simulink model "ClassDMain"  (R2020a)
settings: Solver=VariableStepAuto  StartTime=0.0  StopTime=1  MaxStep=1e-5  RelTol=1e-3
libraries: powerlib x33, dsparch4 x6, powerlib_meascontrol x6, simulink x2
settings Model: Creator=burmesdani  LastModifiedBy=Keshav
settings SolverCC: ZeroCrossAlgorithm=Adaptive
settings DataIOCC: ReturnWorkspaceOutputs=off
settings DebuggingCC: IgnoredZcDiagnostic=none  ArithmeticOperatorsInVariantConditions=warning
settings SFSimCC: SimUseLocalCustomCode=off  CustomCodeUndefinedFunction=UseInterfaceOnly
settings RTWCC: RTWUseLocalCustomCode=off

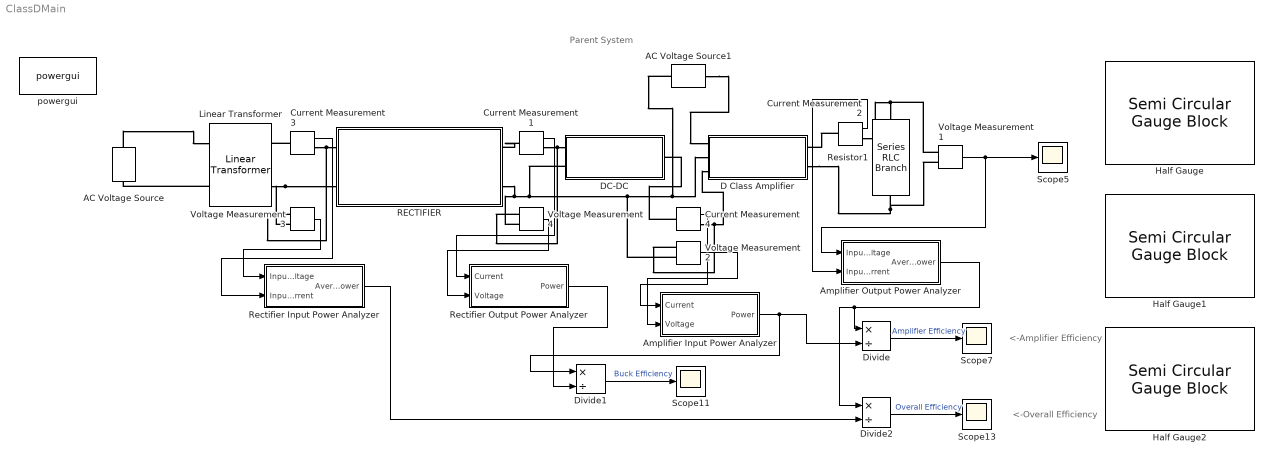
== system ClassDMain ==
  note: Parent System
  note: <-Overall Efficiency
  note: <-Amplifier Efficiency
  AC Voltage Source : powerlib/Electrical Sources/AC Voltage Source  Amplitude=240*sqrt(2)  Phase=0  Frequency=50  SampleTime=0  Measurements=None  BusType=swing  Pref=10e3  Qref=0  Qmin=-inf  Qmax=+inf
  AC Voltage Source1 : powerlib/Electrical Sources/AC Voltage Source  Amplitude=1  Phase=0  Frequency=100  SampleTime=0  Measurements=None  BusType=swing  Pref=10e3  Qref=0  Qmin=-inf  Qmax=+inf
  Amplifier Input Power Analyzer : Subsystem
  Amplifier Output Power Analyzer : Subsystem
  Current Measurement{1..4} (4 alike) : powerlib/Measurements/Current Measurement  PhasorSimulation=off  OutputType=Complex  PSBequivalent=0
  D Class Amplifier : Subsystem  mask{mxsw=1, Fts=2000}
      mask prompts: mxsw "Max input swing"; Fts "Switching Freq"
  DC-DC : Subsystem  mask{Fts=40000, opv=26}
      mask prompts: Fts "SwitchingFreq"; opv "OutputVoltage"
  Divide : Product  Inputs=*/
  Divide1 : Product  Inputs=*/
  Divide2 : Product  Inputs=*/
  Half Gauge : SemiCircularGaugeBlock  ScaleMax=1
  Half Gauge1 : SemiCircularGaugeBlock  ScaleMax=1
  Half Gauge2 : SemiCircularGaugeBlock  ScaleMax=1
  Linear Transformer : powerlib/Elements/Linear Transformer  UNITS=pu  NominalPower=[ 250e6 60 ]  winding1="[ 240  0.002  0.08 ]"  winding2="[ 60  0.002  0.08 ]"  ThreeWindings=off  winding3=[ 315e3 0.002 0.08 ]  RmLm=[ 500 500 ]  Measurements=None  DataType=off
  RECTIFIER : Subsystem
  Rectifier Input Power Analyzer : Subsystem
  Rectifier Output Power Analyzer : Subsystem
  Resistor1 : powerlib/Elements/Series RLC Branch  LConnTagsString=__new0  RConnTagsString=__new0  BranchType=R  Resistance=4  Inductance=1e-3  SetiL0=off  InitialCurrent=0  Capacitance=100e-6  Setx0=off  InitialVoltage=0  Measurements=None
  Scope{5,7,11,13} (4 alike) : Scope
  Voltage Measurement{1..4} (4 alike) : powerlib/Measurements/Voltage Measurement  PhasorSimulation=off  OutputType=Magnitude  PSBequivalent=0
  powergui : powerlib/powergui  Priority=1  SimulationMode=Continuous  SampleTime=50e-6  frequency=60  Iterations=50  frequencyindice=100  Pbase=100e6  ErrMax=1e-4  UnitsV=kV  UnitsW=MW  buscounter=0  FunctionMessages=off  echomessages=off  EnableUseOfTLC=off  CurrentSourceSwitches=off  DisableSnubberDevices=off  DisableRonSwitches=off  DisableVfSwitches=off  DisplayEquations=off  AutomaticDiscreteSolvers=off  SolverType=Tustin/Backward Euler (TBE)  Interpol=off  ExternalGateDelay=off  methode=off  Ts=100  x0status=blocks  SPID=on  SwTol=0  HookPort=off  NonlinearTolerance=1e-4  nMaxIteration=100  ContinueOnMaxIteration=off  RestoreLinks=warning  ResistiveCurrentMeasurement=off  Frange=[0:2:500]  Ylog=off  Xlog=on  ShowGrid=off  save=off  variable=ZData  structure=0  ZoomFFT=off  StartTime=0.0  cycles=1  DisplayStyle=1  fundamental=60  FreqAxis=off  MaxFrequency=1000  frequencyindicesteady=1  RmsSteady=1  display=off
  wires:
  Divide/1 -> Scope7/1  "Amplifier Efficiency"
  Divide1/1 -> Scope11/1  "Buck Efficiency"
  Divide2/1 -> Scope13/1  "Overall Efficiency"
  Voltage Measurement3/1 -> Rectifier Input Power Analyzer/1(Input Voltage)
  Current Measurement3/1 -> Rectifier Input Power Analyzer/2(Input Current)
  Current Measurement1/1 -> Rectifier Output Power Analyzer/1(Current)
  Voltage Measurement4/1 -> Rectifier Output Power Analyzer/2(Voltage)
  Current Measurement4/1 -> Amplifier Input Power Analyzer/1(Current)
  Voltage Measurement2/1 -> Amplifier Input Power Analyzer/2(Voltage)
  Voltage Measurement1/1 -> Scope5/1, Amplifier Output Power Analyzer/1(Input Voltage)
  Current Measurement2/1 -> Amplifier Output Power Analyzer/2(Input Current)
  Rectifier Input Power Analyzer/1(Average power) -> Divide2/2
  Amplifier Output Power Analyzer/1(Average power) -> Divide/1, Divide2/1
  Amplifier Input Power Analyzer/1(Power) -> Divide1/1, Divide/2
  Rectifier Output Power Analyzer/1(Power) -> Divide1/2
  connections:
  Linear Transformer/RConn2 -- RECTIFIER/LConn2 -- Voltage Measurement3/LConn2
  Linear Transformer/LConn2 -- AC Voltage Source/LConn1
  AC Voltage Source/RConn1 -- Linear Transformer/LConn1
  RECTIFIER/RConn2 -- D Class Amplifier/LConn2 -- AC Voltage Source1/LConn1 -- Voltage Measurement2/LConn2 -- DC-DC/LConn2 -- Voltage Measurement4/LConn2
  Current Measurement1/RConn1 -- Voltage Measurement4/LConn1 -- DC-DC/LConn1
  Current Measurement1/LConn1 -- RECTIFIER/RConn1
  AC Voltage Source1/RConn1 -- D Class Amplifier/LConn1
  D Class Amplifier/RConn2 -- Voltage Measurement1/LConn2 -- Resistor1/RConn1
  Current Measurement2/LConn1 -- D Class Amplifier/RConn1
  Current Measurement2/RConn1 -- Voltage Measurement1/LConn1 -- Resistor1/LConn1
  Current Measurement4/RConn1 -- Voltage Measurement2/LConn1 -- D Class Amplifier/LConn3
  Current Measurement4/LConn1 -- DC-DC/RConn1
  Current Measurement3/LConn1 -- Linear Transformer/RConn1
  Current Measurement3/RConn1 -- Voltage Measurement3/LConn1 -- RECTIFIER/LConn1

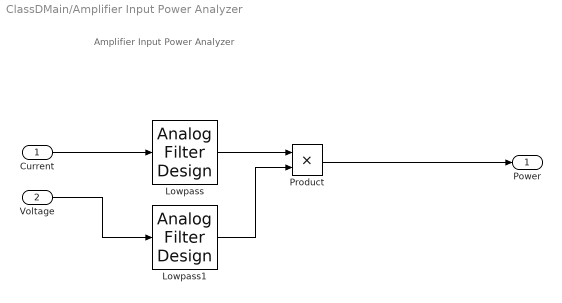
== system ClassDMain/Amplifier Input Power Analyzer ==
  note: Amplifier Input Power Analyzer
  Current : Inport
  Voltage : Inport  Port=2
  Lowpass : dsparch4/Analog Filter Design  method=Butterworth  filttype=Lowpass  N=8  Wlo=200  Whi=80  Rp=1  Rs=40
  Lowpass1 : dsparch4/Analog Filter Design  method=Butterworth  filttype=Lowpass  N=8  Wlo=200  Whi=80  Rp=1  Rs=40
  Product : Product
  Power : Outport
  wires:
  Current/1 -> Lowpass/1
  Lowpass/1 -> Product/1
  Product/1 -> Power/1
  Lowpass1/1 -> Product/2
  Voltage/1 -> Lowpass1/1

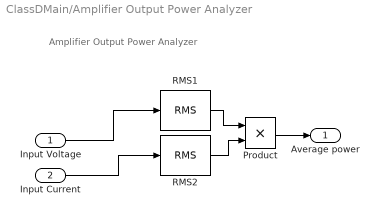
== system ClassDMain/Amplifier Output Power Analyzer ==
  note: Amplifier Output Power Analyzer
  Input Voltage : Inport
  Input Current : Inport  Port=2
  Product : Product
  RMS1 : powerlib_meascontrol/Measurements/RMS  TrueRMS=on  Freq=200  RMSInit=0  Ts=0
  RMS2 : powerlib_meascontrol/Measurements/RMS  TrueRMS=on  Freq=200  RMSInit=0  Ts=0
  Average power : Outport
  wires:
  Product/1 -> Average power/1
  Input Voltage/1 -> RMS1/1
  RMS1/1 -> Product/1
  RMS2/1 -> Product/2
  Input Current/1 -> RMS2/1

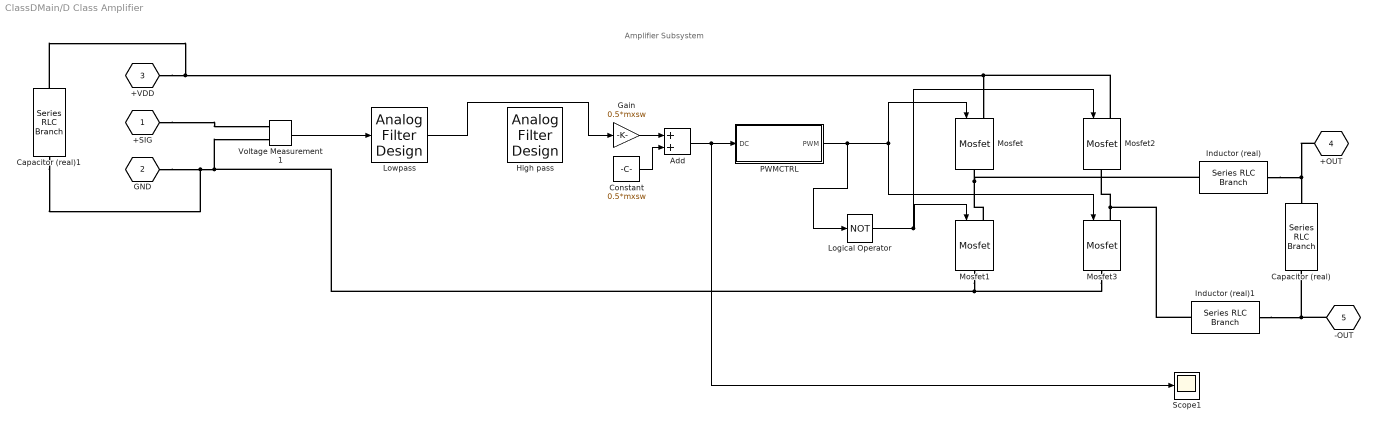
== system ClassDMain/D Class Amplifier ==
  note: Amplifier Subsystem
  Add : Sum
  Capacitor (real) : powerlib/Elements/Series RLC Branch  LConnTagsString=__new0  RConnTagsString=__new0  BranchType=RC  Resistance=0.2  Inductance=1e-3  SetiL0=off  InitialCurrent=0  Capacitance=160e-6  Setx0=off  InitialVoltage=0  Measurements=None
  Capacitor (real)1 : powerlib/Elements/Series RLC Branch  LConnTagsString=__new0  RConnTagsString=__new0  BranchType=RC  Resistance=0.2  Inductance=1e-3  SetiL0=off  InitialCurrent=0  Capacitance=4.7e-3  Setx0=off  InitialVoltage=0  Measurements=None
  Constant : Constant  Value=0.5*mxsw
  Gain : Gain  Gain=0.5*mxsw
  High pass : dsparch4/Analog Filter Design  method=Chebyshev I  filttype=Highpass  N=8  Wlo=31.4  Whi=80  Rp=1  Rs=40
  Inductor (real) : powerlib/Elements/Series RLC Branch  LConnTagsString=__new0  RConnTagsString=__new0  BranchType=RL  Resistance=0.08  Inductance=1e-3  SetiL0=off  InitialCurrent=0  Capacitance=10e-6  Setx0=off  InitialVoltage=0  Measurements=None
  Inductor (real)1 : powerlib/Elements/Series RLC Branch  LConnTagsString=__new0  RConnTagsString=__new0  BranchType=RL  Resistance=0.08  Inductance=1e-3  SetiL0=off  InitialCurrent=0  Capacitance=10e-6  Setx0=off  InitialVoltage=0  Measurements=None
  Logical Operator : Logic  Operator=NOT  Inputs=1  IconShape=distinctive  AllPortsSameDT=off  OutDataTypeStr=boolean
  Lowpass : dsparch4/Analog Filter Design  method=Chebyshev I  filttype=Lowpass  N=8  Wlo=3000  Whi=80  Rp=1  Rs=40
  Mosfet{,1..3} (4 alike) : powerlib/Power Electronics/Mosfet  Ron=0.1  Lon=0  Rd=0.01  Vfd=0  IC=0  Rs=1e5  Cs=inf  Measurements=off
  PWMCTRL : Subsystem  mask{Ft=Fts}
      mask prompts: Ft "Switching Freq"
  Scope1 : Scope
  Voltage Measurement1 : powerlib/Measurements/Voltage Measurement  PhasorSimulation=off  OutputType=Magnitude  PSBequivalent=0
      link override source: GotoTag=T38_3671_2614244151095
  +SIG : PMIOPort  Tag=PMCPort  Side=Left
  GND : PMIOPort  Tag=PMCPort  Port=2  Side=Left
  +VDD : PMIOPort  Tag=PMCPort  Port=3  Side=Left
  +OUT : PMIOPort  Tag=PMCPort  Port=4  Side=Right
  -OUT : PMIOPort  Tag=PMCPort  Port=5  Side=Right
  wires:
  Voltage Measurement1/1 -> Lowpass/1
  Gain/1 -> Add/1
  Constant/1 -> Add/2
  Add/1 -> Scope1/1, PWMCTRL/1(DC)
  PWMCTRL/1(PWM) -> Logical Operator/1, Mosfet3/1, Mosfet/1
  Logical Operator/1 -> Mosfet2/1, Mosfet1/1
  Lowpass/1 -> Gain/1
  connections:
  +SIG/RConn1 -- Voltage Measurement1/LConn1
  GND/RConn1 -- Mosfet3/RConn1 -- Mosfet1/RConn1 -- Voltage Measurement1/LConn2 -- Capacitor (real)1/RConn1
  +VDD/RConn1 -- Capacitor (real)1/LConn1 -- Mosfet2/LConn1 -- Mosfet/LConn1
  Mosfet1/LConn1 -- Inductor (real)/RConn1 -- Mosfet/RConn1
  Mosfet3/LConn1 -- Mosfet2/RConn1 -- Inductor (real)1/RConn1
  Inductor (real)/LConn1 -- Capacitor (real)/LConn1 -- +OUT/RConn1
  -OUT/RConn1 -- Inductor (real)1/LConn1 -- Capacitor (real)/RConn1

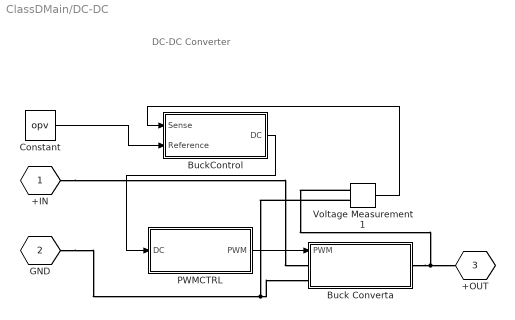
== system ClassDMain/DC-DC ==
  note: DC-DC Converter
  Buck Converta : Subsystem
  BuckControl : Subsystem
  Constant : Constant  Value=opv
  PWMCTRL : Subsystem  mask{Ft=Fts}
      mask prompts: Ft "Switching Freq"
  Voltage Measurement1 : powerlib/Measurements/Voltage Measurement  PhasorSimulation=off  OutputType=Magnitude  PSBequivalent=0
  +IN : PMIOPort  Tag=PMCPort  Side=Left
  GND : PMIOPort  Tag=PMCPort  Port=2  Side=Left
  +OUT : PMIOPort  Tag=PMCPort  Port=3  Side=Right
  wires:
  PWMCTRL/1(PWM) -> Buck Converta/1(PWM)
  BuckControl/1(DC) -> PWMCTRL/1(DC)
  Constant/1 -> BuckControl/2(Reference)
  Voltage Measurement1/1 -> BuckControl/1(Sense)
  connections:
  +IN/RConn1 -- Buck Converta/LConn1
  GND/RConn1 -- Voltage Measurement1/LConn2 -- Buck Converta/LConn2
  Buck Converta/RConn1 -- Voltage Measurement1/LConn1 -- +OUT/RConn1

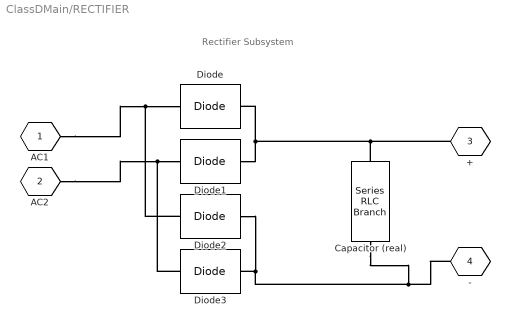
== system ClassDMain/RECTIFIER ==
  note: Rectifier Subsystem
  Capacitor (real) : powerlib/Elements/Series RLC Branch  LConnTagsString=__new0  RConnTagsString=__new0  BranchType=RC  Resistance=0.05  Inductance=1e-3  SetiL0=off  InitialCurrent=0  Capacitance=10e-3  Setx0=off  InitialVoltage=0  Measurements=None
  Diode{,1..3} (4 alike) : powerlib/Power Electronics/Diode  Ron=0.001  Lon=0  Vf=0.8  IC=0  UseSnubber=0  Rs=500  Cs=250e-9  Measurements=off
  AC1 : PMIOPort  Tag=PMCPort  Side=Left
  AC2 : PMIOPort  Tag=PMCPort  Port=2  Side=Left
  + : PMIOPort  Tag=PMCPort  Port=3  Side=Right
  - : PMIOPort  Tag=PMCPort  Port=4  Side=Right
  connections:
  AC1/RConn1 -- Diode2/RConn1 -- Diode/LConn1
  AC2/RConn1 -- Diode3/RConn1 -- Diode1/LConn1
  Diode1/RConn1 -- +/RConn1 -- Capacitor (real)/LConn1 -- Diode/RConn1
  Diode2/LConn1 -- Capacitor (real)/RConn1 -- -/RConn1 -- Diode3/LConn1

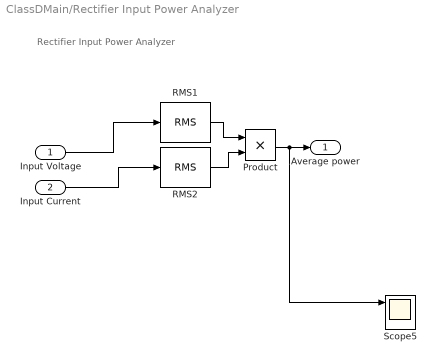
== system ClassDMain/Rectifier Input Power Analyzer ==
  note: Rectifier Input Power Analyzer
  Input Voltage : Inport
  Input Current : Inport  Port=2
  Product : Product
  RMS1 : powerlib_meascontrol/Measurements/RMS  TrueRMS=on  Freq=50  RMSInit=0  Ts=0
  RMS2 : powerlib_meascontrol/Measurements/RMS  TrueRMS=on  Freq=50  RMSInit=0  Ts=0
  Scope5 : Scope  NumInputPorts=3
  Average power : Outport
  wires:
  Product/1 -> Scope5/1, Average power/1
  Input Voltage/1 -> RMS1/1
  RMS1/1 -> Product/1
  RMS2/1 -> Product/2
  Input Current/1 -> RMS2/1

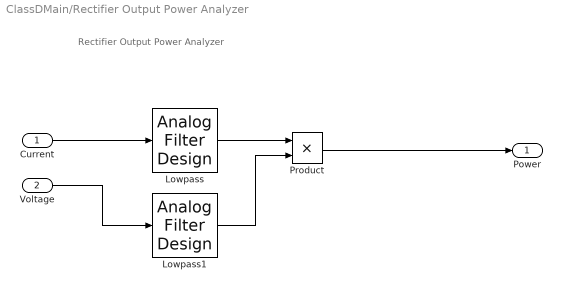
== system ClassDMain/Rectifier Output Power Analyzer ==
  note: Rectifier Output Power Analyzer
  Current : Inport
  Voltage : Inport  Port=2
  Lowpass : dsparch4/Analog Filter Design  method=Butterworth  filttype=Lowpass  N=8  Wlo=200  Whi=80  Rp=1  Rs=40
  Lowpass1 : dsparch4/Analog Filter Design  method=Butterworth  filttype=Lowpass  N=8  Wlo=200  Whi=80  Rp=1  Rs=40
  Product : Product
  Power : Outport
  wires:
  Current/1 -> Lowpass/1
  Lowpass/1 -> Product/1
  Product/1 -> Power/1
  Lowpass1/1 -> Product/2
  Voltage/1 -> Lowpass1/1

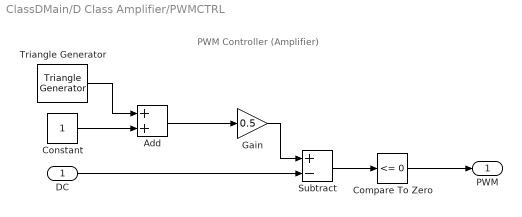
== system ClassDMain/D Class Amplifier/PWMCTRL ==
  note: PWM Controller (Amplifier)
  DC : Inport
  Add : Sum
  Compare To Zero : simulink/Logic and Bit Operations/Compare To Zero  relop=<=  OutDataTypeStr=boolean
  Constant : Constant
  Gain : Gain  Gain=0.5
  Subtract : Sum  Inputs=+-
  Triangle Generator : powerlib_meascontrol/Pulse & Signal Generators/Triangle Generator  Freq=Ft  Phase=90  Ts=0
  PWM : Outport
  wires:
  Triangle Generator/1 -> Add/1
  Constant/1 -> Add/2
  Add/1 -> Gain/1
  Gain/1 -> Subtract/1
  DC/1 -> Subtract/2
  Subtract/1 -> Compare To Zero/1
  Compare To Zero/1 -> PWM/1

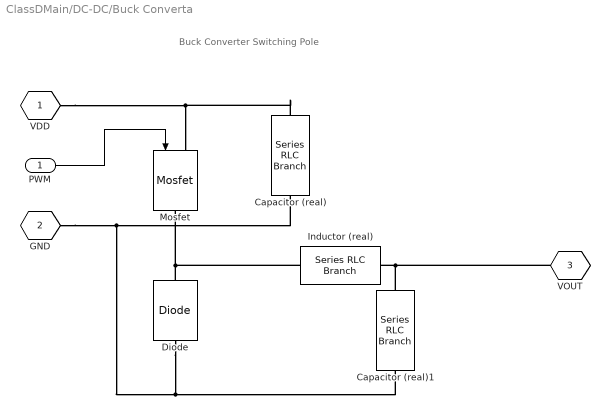
== system ClassDMain/DC-DC/Buck Converta ==
  note: Buck Converter Switching Pole
  PWM : Inport
  Capacitor (real) : powerlib/Elements/Series RLC Branch  LConnTagsString=__new0  RConnTagsString=__new0  BranchType=RC  Resistance=0.05  Inductance=1e-3  SetiL0=off  InitialCurrent=0  Capacitance=10e-6  Setx0=off  InitialVoltage=0  Measurements=None
  Capacitor (real)1 : powerlib/Elements/Series RLC Branch  LConnTagsString=__new0  RConnTagsString=__new0  BranchType=RC  Resistance=0.05  Inductance=1e-3  SetiL0=off  InitialCurrent=0  Capacitance=300e-6  Setx0=off  InitialVoltage=0  Measurements=None
  Diode : powerlib/Power Electronics/Diode  Ron=0.001  Lon=0  Vf=0.8  IC=0  UseSnubber=0  Rs=500  Cs=250e-9  Measurements=off
  Inductor (real) : powerlib/Elements/Series RLC Branch  LConnTagsString=__new0  RConnTagsString=__new0  BranchType=RL  Resistance=0.08  Inductance=390e-6  SetiL0=off  InitialCurrent=0  Capacitance=10e-6  Setx0=off  InitialVoltage=0  Measurements=None
  Mosfet : powerlib/Power Electronics/Mosfet  Ron=0.1  Lon=0  Rd=0.01  Vfd=0  IC=0  Rs=1e5  Cs=inf  Measurements=off
  VDD : PMIOPort  Tag=PMCPort  Side=Left
  GND : PMIOPort  Tag=PMCPort  Port=2  Side=Left
  VOUT : PMIOPort  Tag=PMCPort  Port=3  Side=Right
  wires:
  PWM/1 -> Mosfet/1
  connections:
  Capacitor (real)/LConn1 -- VDD/RConn1 -- Mosfet/LConn1
  Inductor (real)/RConn1 -- Diode/RConn1 -- Mosfet/RConn1
  Capacitor (real)1/LConn1 -- VOUT/RConn1 -- Inductor (real)/LConn1
  Capacitor (real)/RConn1 -- GND/RConn1 -- Capacitor (real)1/RConn1 -- Diode/LConn1

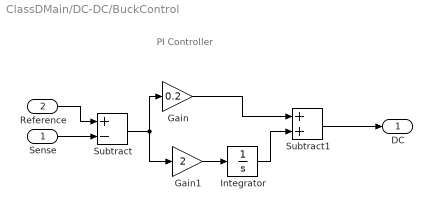
== system ClassDMain/DC-DC/BuckControl ==
  note: PI Controller
  Sense : Inport
  Reference : Inport  Port=2
  Gain : Gain  Gain=0.2
  Gain1 : Gain  Gain=2
  Integrator : Integrator  ZeroCross=off
  Subtract : Sum  Inputs=+-
  Subtract1 : Sum
  DC : Outport
  wires:
  Sense/1 -> Subtract/2
  Reference/1 -> Subtract/1
  Subtract/1 -> Gain1/1, Gain/1
  Gain1/1 -> Integrator/1
  Integrator/1 -> Subtract1/2
  Subtract1/1 -> DC/1
  Gain/1 -> Subtract1/1

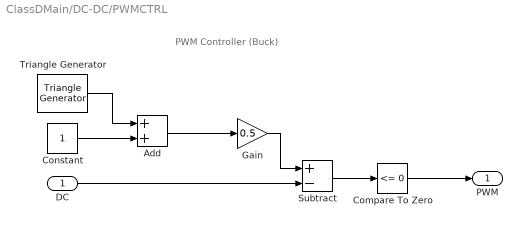
== system ClassDMain/DC-DC/PWMCTRL ==
  note: PWM Controller (Buck)
  DC : Inport
  Add : Sum
  Compare To Zero : simulink/Logic and Bit Operations/Compare To Zero  relop=<=  OutDataTypeStr=boolean
  Constant : Constant
  Gain : Gain  Gain=0.5
  Subtract : Sum  Inputs=+-
  Triangle Generator : powerlib_meascontrol/Pulse & Signal Generators/Triangle Generator  Freq=Ft  Phase=90  Ts=0
  PWM : Outport
  wires:
  Triangle Generator/1 -> Add/1
  Constant/1 -> Add/2
  Add/1 -> Gain/1
  Gain/1 -> Subtract/1
  DC/1 -> Subtract/2
  Subtract/1 -> Compare To Zero/1
  Compare To Zero/1 -> PWM/1
